simulink model "Exp1_pendulum"  (R2023b)
settings: Solver=ode3  StartTime=0.0  StopTime=2000.0  FixedStep=0.001  RelTol=1e-3
undefined symbols (not defined in the file): d, Fgl, J, omega_0, phi_0
settings Model: Creator=tunkarlu  LastModifiedBy=tunkarlu

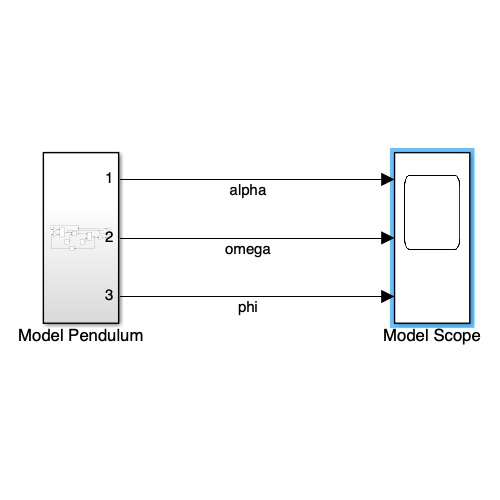
[thumbnail: Simulink's stored preview of the top-level diagram]
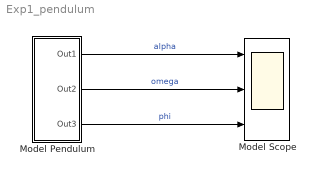
== system Exp1_pendulum ==
  Model Pendulum : Subsystem
  Model Scope : Scope  NumInputPorts=3
  wires:
  Model Pendulum/1(Out1) -> Model Scope/1  "alpha"
  Model Pendulum/2(Out2) -> Model Scope/2  "omega"
  Model Pendulum/3(Out3) -> Model Scope/3  "phi"

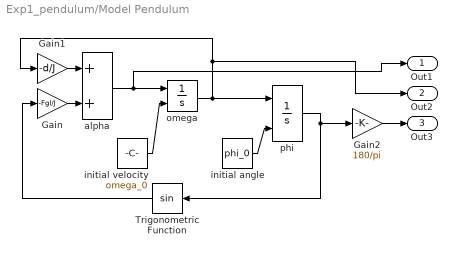
== system Exp1_pendulum/Model Pendulum ==
  Gain : Gain  Gain=-Fgl/J
  Gain1 : Gain  Gain=-d/J
  Gain2 : Gain  Gain=180/pi
  Trigonometric Function : Trigonometry
  alpha : Sum
  initial angle : Constant  Value=phi_0
  initial velocity : Constant  Value=omega_0
  omega : Integrator  InitialConditionSource=external
  phi : Integrator  InitialConditionSource=external
  Out1 : Outport
  Out2 : Outport  Port=2
  Out3 : Outport  Port=3
  wires:
  Gain/1 -> alpha/2
  Trigonometric Function/1 -> Gain/1
  alpha/1 -> Out1/1, omega/1
  initial velocity/1 -> omega/2
  Gain1/1 -> alpha/1
  initial angle/1 -> phi/2
  phi/1 -> Gain2/1, Trigonometric Function/1
  omega/1 -> Gain1/1, Out2/1, phi/1
  Gain2/1 -> Out3/1
